simulink model "Wind_Turbine_test"  (R2023b)
settings: Solver=VariableStepAuto  StartTime=0.0  StopTime=1  RelTol=1e-3
model workspace (MAT data in the model file):
  Compensation_Ki = 30
  Compensation_Kp = 3
  DC_Ki = 400
  DC_Kp = 8
  F = 0.01
  Flux_min = 0.5
  Grid_Freq_PWM = 2700
  Grid_Ireg_Ki = 5
  Grid_Ireg_Kp = 0.83
  Grid_Ireg_lim = 1.1
  Grid_Modindex_Upper = 1.1
  Grid_conv_Imax = 0.8
  H = 0.685
  Idref_max = 0.9
  Iqref_Tc = 0.3
  Ki_Var = 0.05
  Ki_Vreg = 20
  Ksh = 1.1
  L_pu = 0.3
  Llr = 0.16
  Lls = 0.18
  Lm = 2.9
  P_mech = 1080000
  Pitch_Ki = 0
  Pitch_Kp = 150
  Pitch_Max = 27
  Pitch_Tc = 0.01
  Pitch_rate = 10
  Q_Filt = 50
  R_pu = 0.003
  Rotor_Freq_PWM = 1620
  Rotor_Ireg_Ki = 8
  Rotor_Ireg_Kp = 0.6
  Rotor_Ireg_lim = 0.1
  Rotor_Modindex_Upper = 2
  Rr = 0.016
  Rs = 0.023
  T_set = 0.0001
  Tp = 5e-05
  Ts = 5e-06
  Var_C_Filt = 720000
  Var_reg_max = 1.1
  Var_reg_min = 0.9
  WT_Coeff = [0.645 116 0.4 5 21 0.00912 0.08 0.035]
  WT_H = 4.32
  WT_IGBTRon = 5.931
  WT_Param = [91.204 10143]
  Wind_Freq_Filt = 10000
  Wind_Freq_nom = 60
  Wind_P_nom = 1200000
  Wind_Rotor_V_nom = 1950
  Wind_V_nom = 500
  Zeta_Filt = 0.707106781187
  init = [-0.2 0 0 0 0 0 0 0]
  p = 3
  torque0 = 0.83
  v_Ki = 0.1
  v_Kp = 3.6
  v_Max = 1.2
  v_Min = 0.7
  v_T = 5
  vreg_max = 1
  wind_VDC_nom = 1150
  wt0 = 1.2
undefined symbols (not defined in the file): D1, D11, Delta, DiscIntNeverNeededParam, P, Q
libraries: powerlib_extras x144, simulink_extras x24, spsThreePhaseVIMeasurementLib x13, spsThreePhaseTransformerTwoWindingsLib x11, spsSeriesRLCBranchLib x9, spsPWMGenerator2LevelLib x8, spsUniversalBridgeLib x8, spsThreePhaseSeriesRLCLoadLib x6, spsThreePhasePISectionLineLib x5, spsGroundLib x5, spsLoadFlowBusLib x4, spsAsynchronousMachinepuUnitsLib x4
(part 3 of 9)

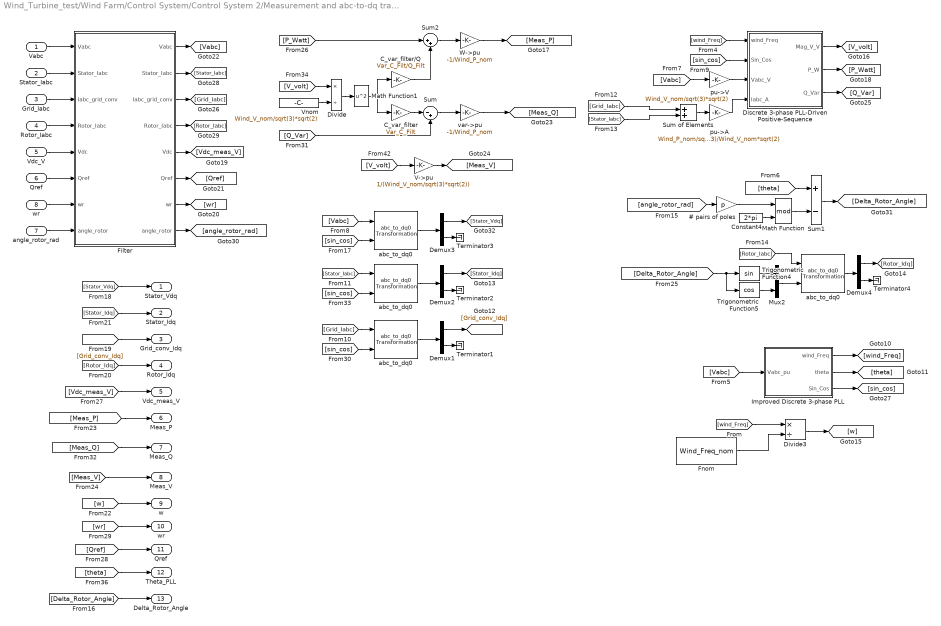
== system Wind_Turbine_test/Wind Farm/Control System/Control System 2/Measurement and abc-to-dq transformation  ==
  Vabc : Inport
  Stator_Iabc : Inport  Port=2
  Grid_Iabc : Inport  Port=3
  Rotor_Iabc : Inport  Port=4
  Vdc_V : Inport  Port=5
  Qref : Inport  Port=6
  angle_rotor_rad : Inport  Port=7
  wr : Inport  Port=8
  "   abc_to_dq0    " : powerlib_extras/Measurements/abc_to_dq0 Transformation
  " Improved Discrete 3-phase PLL" : Subsystem  mask(Discrete 3-phase PLL){Fmin=0.75*Wind_Freq_nom, Par_Init=[0 Wind_Freq_nom], ParK=[5 3.2 1 50], Ts=Ts}
      mask prompts: Fmin "Minimum frequency (Hz):"; Par_Init "Initial inputs:[ Phase(degrees)   Frequency(Hz) ]"; ParK "Regulator gains [ Kp1 Kp2  Ki1  Ki2 ]"; Ts "Sample time:"
      mask help:
      | This Phase Locked Loop (PLL) system can be used  to synchronize on a set of variable frequency, three-phase sinusoidal signals.
      |
      | Input 1: Vector containing the normalized
      |              three-phase signals [Va Vb Vc]
      | Output 1:  Measured frequency (Hz) = w/(2pi)
      | Output 2:  Ramp w.t   varying between  0 and 2*pi,
      | synchronized on zero crossings of the fundamental (positive-sequence) of phase A.
      | Output 3: Vector [sin(wt) cos(wt)]
      mask init:
      | Kp1=ParK(1);
      | Kp2=ParK(2);
      | Ki1=ParK(3);
      | Ki2=ParK(4);
      | Phase_Init=Par_Init(1);
      | Finit=Par_Init(2);
      | power_initmask();
      settings: OpenFcn=power_openblockproxy();
  # pairs of poles : Gain  Gain=p  SaturateOnIntegerOverflow=on  OutDataTypeStr=Inherit: Same as input  ParamDataTypeStr=Inherit: Same as input
  C_var_filter : Gain  Gain=Var_C_Filt  SaturateOnIntegerOverflow=on  OutDataTypeStr=Inherit: Same as input  ParamDataTypeStr=Inherit: Same as input
  C_var_filter/Q : Gain  Gain=Var_C_Filt/Q_Filt  SaturateOnIntegerOverflow=on  OutDataTypeStr=Inherit: Same as input  ParamDataTypeStr=Inherit: Same as input
  Constant4 : Constant  Value=2*pi
  Demux{1..4} (4 alike) : Demux  Outputs=[2 1]
      settings: DisplayOption=none
  "Discrete 3-phase PLL-Driven Positive-Sequence " : Subsystem  mask(Discrete 3-phase PLL-Driven Positive-Sequence Active & Reactive Power){Finit=Wind_Freq_nom, Fmin=Wind_Freq_nom*45/60, Par_Vinit=[Wind_V_nom/sqrt(3)*sqrt(2) 30], Par_Iinit=[Wind_P_nom/sqrt(3)/Wind_V_nom*sqrt(2) -10], Ts=Ts}
      mask prompts: Finit "Initial frequency (Hz):"; Fmin "Minimum frequency (Hz):"; Par_Vinit "Voltage initial input: [ Mag  Phase(Degrees) ]"; Par_Iinit "Current initial input: [ Mag  Phase(Degrees) ]"; Ts "Sample time:"
      mask help:
      | This discrete block measures the 3-phase active power P and reactive power Q  associated with a periodic set of 3-phase voltages and currents which may contain harmonics. P and Q are calculated by evaluating the fundamental values (positive-sequence) of the input voltages and currents with a running window over one cycle of the specified frequency (port Freq).
      |  Input port "Sin_Cos" (a two-dimension signal) provides the reference frame required for the computation.
      |
      | input 1: must give the frequency of the fundamental (Hz)
      | Input 2: must contain a  [sin(wt)  cos(wt)] two dimension signal , where w is the rotation speed (rad/s) of the reference frame used for the computation..
      | input 3: Vectorized 3-phase  instantaneous voltage (Vabc)
      | input 4: Vectorized 3-phase instantaneous current (Iabc)
      |
      | Output 1: Vector [Mag_V Mag_I] of the fundamental values (Magnitude) of the voltage & current (peak values of the positive-sequence)
      | Output 2: 3-phase PQ measurement vector [P(W) Q (var)] evaluated at the specified frequency. Current flowing into an RL circuit will produce  positive active and reactive powers.
      |
      | For the first cycle of simulation, the outputs are held constant using the values specified by the parameters "Initial input".
      | he value of the parameter "Minimum frequency" is used to determine the buffer size of the "Variable Transport Delay" block found inside this subsystem.
      mask init:
      | power_initmask();
      settings: OpenFcn=power_openblockproxy();
  Divide : Product  Inputs=*/
  Divide3 : Product  Inputs=*/
  Filter : Subsystem  mask{Freq=Wind_Freq_Filt, Zeta1=Zeta_Filt, Ts=Ts}
      mask prompts: Freq "Cut-off frequency (Hz):"; Zeta1 "Damping factor Zeta:"; Ts "Sample time"
  Fnom : Constant  Value=Wind_Freq_nom
  Math Function : Math  Operator=mod  SignedPower=on
  Math Function1 : Math  Operator=square  SignedPower=on
  Mux2 : Mux  Inputs=2
  Sum : Sum  Inputs=|-+
  Sum of Elements : Sum
  Sum1 : Sum  Inputs=+-  InputSameDT=on  SaturateOnIntegerOverflow=on  OutDataTypeStr=Inherit: Same as first input
  Sum2 : Sum  Inputs=|++
  Terminator{1..4} (4 alike) : Terminator
  Trigonometric Function4 : Trigonometry
  Trigonometric Function5 : Trigonometry  Operator=cos
  V->pu : Gain  Gain=1/(Wind_V_nom/sqrt(3)*sqrt(2))  SaturateOnIntegerOverflow=on  OutDataTypeStr=Inherit: Same as input  ParamDataTypeStr=Inherit: Same as input
  Vnom : Constant  Value=Wind_V_nom/sqrt(3)*sqrt(2)
  W->pu : Gain  Gain=-1/Wind_P_nom  SaturateOnIntegerOverflow=on  OutDataTypeStr=Inherit: Same as input  ParamDataTypeStr=Inherit: Same as input
  abc_to_dq0 : powerlib_extras/Measurements/abc_to_dq0 Transformation
  "abc_to_dq0 " : powerlib_extras/Measurements/abc_to_dq0 Transformation
  "abc_to_dq0  " : powerlib_extras/Measurements/abc_to_dq0 Transformation
  pu->A : Gain  Gain=Wind_P_nom/sqrt(3)/Wind_V_nom*sqrt(2)  SaturateOnIntegerOverflow=on  OutDataTypeStr=Inherit: Same as input  ParamDataTypeStr=Inherit: Same as input
  pu->V : Gain  Gain=Wind_V_nom/sqrt(3)*sqrt(2)  SaturateOnIntegerOverflow=on  OutDataTypeStr=Inherit: Same as input  ParamDataTypeStr=Inherit: Same as input
  "var->pu " : Gain  Gain=-1/Wind_P_nom  SaturateOnIntegerOverflow=on  OutDataTypeStr=Inherit: Same as input  ParamDataTypeStr=Inherit: Same as input
  Stator_Vdq : Outport  VectorParamsAs1DForOutWhenUnconnected=off
  Stator_Idq : Outport  Port=2  VectorParamsAs1DForOutWhenUnconnected=off
  Grid_conv_Idq : Outport  Port=3  VectorParamsAs1DForOutWhenUnconnected=off
  Rotor_Idq : Outport  Port=4  VectorParamsAs1DForOutWhenUnconnected=off
  Vdc_meas_V : Outport  Port=5  VectorParamsAs1DForOutWhenUnconnected=off
  Meas_P : Outport  Port=6  VectorParamsAs1DForOutWhenUnconnected=off
  Meas_Q : Outport  Port=7  VectorParamsAs1DForOutWhenUnconnected=off
  Meas_V : Outport  Port=8  VectorParamsAs1DForOutWhenUnconnected=off
  w : Outport  Port=9  VectorParamsAs1DForOutWhenUnconnected=off
  "wr " : Outport  Port=10  VectorParamsAs1DForOutWhenUnconnected=off
  "Qref " : Outport  Port=11  VectorParamsAs1DForOutWhenUnconnected=off
  Theta_PLL : Outport  Port=12  VectorParamsAs1DForOutWhenUnconnected=off
  Delta_Rotor_Angle : Outport  Port=13  VectorParamsAs1DForOutWhenUnconnected=off
  wires:
  Math Function/1 -> Sum1/2
  [wind_Freq] -> "Discrete 3-phase PLL-Driven Positive-Sequence "/1(wind_Freq)
  [P_Watt] -> Sum2/1
  [sin_cos] -> abc_to_dq0/2
  [Meas_Q] -> Meas_Q/1
  [Q_Var] -> Sum/2
  Math Function1/1 -> C_var_filter/Q/1, C_var_filter/1
  Sum of Elements/1 -> pu->A/1
  [Grid_Iabc] -> Sum of Elements/1
  [Grid_conv_Idq] -> Grid_conv_Idq/1
  Filter/6("Qref ") -> [Qref]
  W->pu/1 -> [Meas_P]
  [Stator_Idq] -> Stator_Idq/1
  "Discrete 3-phase PLL-Driven Positive-Sequence "/1(Mag_V_V) -> [V_volt]
  Demux1/2 -> Terminator1/1
  [wr] -> "wr "/1
  Filter/3("Iabc_grid_conv ") -> [Grid_Iabc]
  Filter/2("Stator_Iabc ") -> [Stator_Iabc]
  [Meas_P] -> Meas_P/1
  [Delta_Rotor_Angle] -> Trigonometric Function4/1, Trigonometric Function5/1
  Vnom/1 -> Divide/2
  [w] -> w/1
  "var->pu "/1 -> [Meas_Q]
  Sum2/1 -> W->pu/1
  [wind_Freq] -> Divide3/1
  [Delta_Rotor_Angle] -> Delta_Rotor_Angle/1
  Vdc_V/1 -> Filter/5(Vdc)
  "Discrete 3-phase PLL-Driven Positive-Sequence "/3(Q_Var) -> [Q_Var]
  [Vabc] -> pu->V/1
  wr/1 -> Filter/7(wr)
  Fnom/1 -> Divide3/2
  [Vabc] -> " Improved Discrete 3-phase PLL"/1(Vabc_pu)
  "Discrete 3-phase PLL-Driven Positive-Sequence "/2(P_W) -> [P_Watt]
  Trigonometric Function5/1 -> Mux2/2
  [sin_cos] -> "abc_to_dq0 "/2
  [V_volt] -> Divide/1
  Demux3/2 -> Terminator3/1
  Filter/5("Vdc ") -> [Vdc_meas_V]
  Filter/1("Vabc ") -> [Vabc]
  [sin_cos] -> "abc_to_dq0  "/2
  angle_rotor_rad/1 -> Filter/8(angle_rotor)
  "   abc_to_dq0    "/1 -> Demux4/1
  Divide3/1 -> [w]
  Divide/1 -> Math Function1/1
  # pairs of poles/1 -> Math Function/1
  [Stator_Iabc] -> "abc_to_dq0 "/1
  Filter/8("angle_rotor ") -> [angle_rotor_rad]
  Sum/1 -> "var->pu "/1
  [Stator_Vdq] -> Stator_Vdq/1
  Demux4/1 -> [Rotor_Idq]
  [Grid_Iabc] -> "abc_to_dq0  "/1
  [angle_rotor_rad] -> # pairs of poles/1
  Mux2/1 -> "   abc_to_dq0    "/2
  Demux2/2 -> Terminator2/1
  [V_volt] -> V->pu/1
  [Rotor_Iabc] -> "   abc_to_dq0    "/1
  Demux1/1 -> [Grid_conv_Idq]
  Filter/7("wr ") -> [wr]
  [Meas_V] -> Meas_V/1
  [Rotor_Idq] -> Rotor_Idq/1
  Constant4/1 -> Math Function/2
  Demux4/2 -> Terminator4/1
  [sin_cos] -> "Discrete 3-phase PLL-Driven Positive-Sequence "/2(Sin_Cos)
  Qref/1 -> Filter/6(Qref)
  Trigonometric Function4/1 -> Mux2/1
  [Vabc] -> abc_to_dq0/1
  Vabc/1 -> Filter/1(Vabc)
  Rotor_Iabc/1 -> Filter/4(Rotor_Iabc)
  [Qref] -> "Qref "/1
  C_var_filter/Q/1 -> Sum2/2
  Grid_Iabc/1 -> Filter/3(Iabc_grid_conv)
  " Improved Discrete 3-phase PLL"/3(Sin_Cos) -> [sin_cos]
  abc_to_dq0/1 -> Demux3/1
  Stator_Iabc/1 -> Filter/2(Stator_Iabc)
  V->pu/1 -> [Meas_V]
  "abc_to_dq0  "/1 -> Demux1/1
  Demux3/1 -> [Stator_Vdq]
  " Improved Discrete 3-phase PLL"/1(wind_Freq) -> [wind_Freq]
  [theta] -> Theta_PLL/1
  [Vdc_meas_V] -> Vdc_meas_V/1
  Filter/4("Rotor_Iabc ") -> [Rotor_Iabc]
  Sum1/1 -> [Delta_Rotor_Angle]
  "abc_to_dq0 "/1 -> Demux2/1
  [Stator_Iabc] -> Sum of Elements/2
  C_var_filter/1 -> Sum/1
  pu->V/1 -> "Discrete 3-phase PLL-Driven Positive-Sequence "/3(Vabc_V)
  Demux2/1 -> [Stator_Idq]
  [theta] -> Sum1/1
  " Improved Discrete 3-phase PLL"/2(theta) -> [theta]
  pu->A/1 -> "Discrete 3-phase PLL-Driven Positive-Sequence "/4(Iabc_A)

== system Wind_Turbine_test/Wind Farm/Control System/Control System 2/Rotor-side Control System ==
  Rotor_Idq : Inport
  wr : Inport  Port=2
  Vdc : Inport  Port=3
  Angle : Inport  Port=4
  Qref : Inport  Port=5
  Meas_Q : Inport  Port=6
  Meas_V : Inport  Port=7
  Stator_Vdq : Inport  Port=8
  w : Inport  Port=9
  Stator_Idq : Inport  Port=10
  Tem_cmd : Inport  Port=11
  Current Regulator : Subsystem
  "Electromagnetic Torque Controller " : Subsystem
  Gain : Gain  Gain=-1
  "Iqr, ref_limit" : Subsystem
  Modulation Index & Phase : Subsystem
  Rotor Control Voltage Converter : Subsystem
  Var Regulator : Subsystem
  Voltage Regulator : Subsystem
  Uctrl_rotor_conv : Outport  VectorParamsAs1DForOutWhenUnconnected=off
  wires:
  "Electromagnetic Torque Controller "/1(Rotor_Id_ref) -> Current Regulator/1(Rotor_Id_ref), "Iqr, ref_limit"/1(Rotor_Id_ref)
  Qref/1 -> Var Regulator/1(Qref)
  Meas_Q/1 -> Var Regulator/2(Meas_Q)
  Meas_V/1 -> Var Regulator/3(Meas_V)
  "Iqr, ref_limit"/1(Iqrlim) -> Voltage Regulator/1(Max), Gain/1
  Var Regulator/1(Out1) -> Voltage Regulator/3(In)
  Rotor_Idq/1 -> Current Regulator/2(Rotor_Idq)
  wr/1 -> Current Regulator/4(wr)
  Voltage Regulator/1(Iqr_ref) -> Current Regulator/3(Iqr_ref)
  Angle/1 -> Rotor Control Voltage Converter/3(Angle)
  Rotor Control Voltage Converter/1(Uctrl_rotor_conv) -> Uctrl_rotor_conv/1
  Vdc/1 -> Modulation Index & Phase/3(Vdc)
  Modulation Index & Phase/1(x1) -> Rotor Control Voltage Converter/1(x1)
  Modulation Index & Phase/2(y1) -> Rotor Control Voltage Converter/2(y1)
  Current Regulator/1(Rotor_conv_Vd) -> Modulation Index & Phase/1(x)
  Current Regulator/2(Rotor_conv_Vq) -> Modulation Index & Phase/2(y)
  Stator_Vdq/1 -> "Electromagnetic Torque Controller "/1(Stator_Vdq)
  w/1 -> "Electromagnetic Torque Controller "/2(w)
  Stator_Idq/1 -> "Electromagnetic Torque Controller "/3(Stator_Idq)
  Tem_cmd/1 -> "Electromagnetic Torque Controller "/4(Tem_cmd)
  Gain/1 -> Voltage Regulator/2(Min)

== system Wind_Turbine_test/Wind Farm/Control System/Control System 2/Speed & Pitch Control System ==
  wr1 : Inport
  Meas_P : Inport  Port=2
  0-inf : Saturate  UpperLimit=inf  LowerLimit=0
  0-pitch_max : Saturate  UpperLimit=Pitch_Max  LowerLimit=0
  "0-pitch_max " : Saturate  UpperLimit=Pitch_Max  LowerLimit=0
  Constant2 : Constant
  Discrete PI Controller : Subsystem  DialogController=POWERSYS.PowerSysDialog  mask(Discrete PI Controller){Kp=v_Kp, Ki=v_Ki, Par_Limits=[vreg_max 0], Init=0.7, Ts=Ts}
      mask prompts: Kp "Proportional gain (Kp):"; Ki "Integral gain (Ki):"; Par_Limits "Output limits: [ Upper   Lower ]"; Init "Output initial value:"; Ts "Sample time:"
      mask help: This block implements a discrete PI controller.
      mask init:
      | UpperLimit=Par_Limits(1);
      | LowerLimit=Par_Limits(2);
      | power_initmask();
      mask Help: This block is part of a subset of blocks in the Extras library that does not have documentation associated with it, other than the block mask description.
      mask Display: disp('PI');
  Discrete PI Controller1 : powerlib_extras/Discrete  Control Blocks/Discrete PI Controller  Kp=Compensation_Kp  Ki=Compensation_Ki  Par_Limits=[Pitch_Max 0]  Init=0  Ts=Ts
  Gain2 : Gain  Gain=Pitch_Kp  SaturateOnIntegerOverflow=on  OutDataTypeStr=Inherit: Same as input  ParamDataTypeStr=Inherit: Same as input
  Rate Limiter   1 : RateLimiter  RisingSlewLimit=Pitch_rate  FallingSlewLimit=-Pitch_rate
  Saturation : Saturate  UpperLimit=v_Max  LowerLimit=v_Min
  Sum : Sum  Inputs=-+  SaturateOnIntegerOverflow=on
  Sum1 : Sum  Inputs=|+-
  Sum2 : Sum  Inputs=|+-  SaturateOnIntegerOverflow=on
  Sum3 : Sum  Inputs=|++
  Switch : Switch  Threshold=0.75  SaturateOnIntegerOverflow=off  InputSameDT=off
  Tracking Curve : Fcn  Expr=-0.67*u(1)^2+1.42*u(1)+0.51
  pu_elec->pu_mec : Gain  Gain=Wind_P_nom/P_mech
  t=Pitch_time_constant : powerlib_extras/Discrete  Control Blocks/Discrete 1st-Order Filter  FilterType=Lowpass  Tc=Pitch_Tc  Ts=Ts  Initialize=on  Vac_Init=[0.8 -25 60]*0  Vdc_Init=0  PlotResponse=off  param1=[1 500 0.1]
  t=T_speed : powerlib_extras/Discrete  Control Blocks/Discrete 1st-Order Filter  FilterType=Lowpass  Tc=v_T  Ts=Ts  Initialize=on  Vac_Init=[0 0 0]  Vdc_Init=1-init(1)  PlotResponse=off  param1=[1 500 0.1]
  wref : Constant  Value=1.2
  Tem_cmd : Outport  VectorParamsAs1DForOutWhenUnconnected=off
  Pitch (deg) : Outport  Port=2  VectorParamsAs1DForOutWhenUnconnected=off
  wires:
  Rate Limiter   1/1 -> "0-pitch_max "/1
  Switch/1 -> Saturation/1
  Sum3/1 -> Rate Limiter   1/1
  Sum1/1 -> Discrete PI Controller/1(Error)
  Saturation/1 -> t=T_speed/1
  Constant2/1 -> Sum2/2  "Pref"
  Discrete PI Controller1/1 -> Sum3/2
  Meas_P/1 -> 0-inf/1
  t=T_speed/1 -> Sum/1, Sum1/2  "wref"
  0-inf/1 -> pu_elec->pu_mec/1
  wr1/1 -> Sum/2, Sum1/1
  wref/1 -> Switch/1
  0-pitch_max/1 -> Sum3/1
  Discrete PI Controller/1(Out) -> Tem_cmd/1
  t=Pitch_time_constant/1 -> Pitch (deg)/1
  Sum2/1 -> Discrete PI Controller1/1
  Gain2/1 -> 0-pitch_max/1
  pu_elec->pu_mec/1 -> Switch/2, Tracking Curve/1, Sum2/1
  "0-pitch_max "/1 -> t=Pitch_time_constant/1
  Sum/1 -> Gain2/1
  Tracking Curve/1 -> Switch/3

== system Wind_Turbine_test/Wind Farm/Control System/Control System 3/Grid-side Control System ==
  note: Required value for modulation index "m" to obtain 1 pu generated voltage by the converter:
  note: m = Vnom * 2*sqrt(2/3) / Vdc
  note: Where Vnom = RMS ph-ph nominal voltage
  Stator_Vdq : Inport
  Iq_ref : Inport  Port=2
  Vdc : Inport  Port=3
  Grid_conv_Idq : Inport  Port=4
  Theta_PLL : Inport  Port=5
  w : Inport  Port=6
  Current Regulator : Subsystem
  Grid Voltage Converter : Subsystem
  Modulation : Subsystem
  VDC Regulator : Subsystem
  Grid_conv_V : Outport  VectorParamsAs1DForOutWhenUnconnected=off
  wires:
  Current Regulator/1(Grid_conv_Vd) -> Modulation/1(x)
  Current Regulator/2(Grid_conv_Vq) -> Modulation/2(y)
  Grid Voltage Converter/1(Grid_conv_V) -> Grid_conv_V/1
  Theta_PLL/1 -> Grid Voltage Converter/2(Theta_PLL)
  VDC Regulator/1(Out1) -> Current Regulator/2(In2)
  Iq_ref/1 -> VDC Regulator/1(Iq_ref)
  Grid_conv_Idq/1 -> Current Regulator/3(Grid_conv_Idq)
  Stator_Vdq/1 -> Current Regulator/1(Stator_Vdq)
  w/1 -> Current Regulator/4(w)
  Modulation/1(Vdq0) -> Grid Voltage Converter/1(dq0)
  Vdc/1 -> VDC Regulator/2(Vdc)

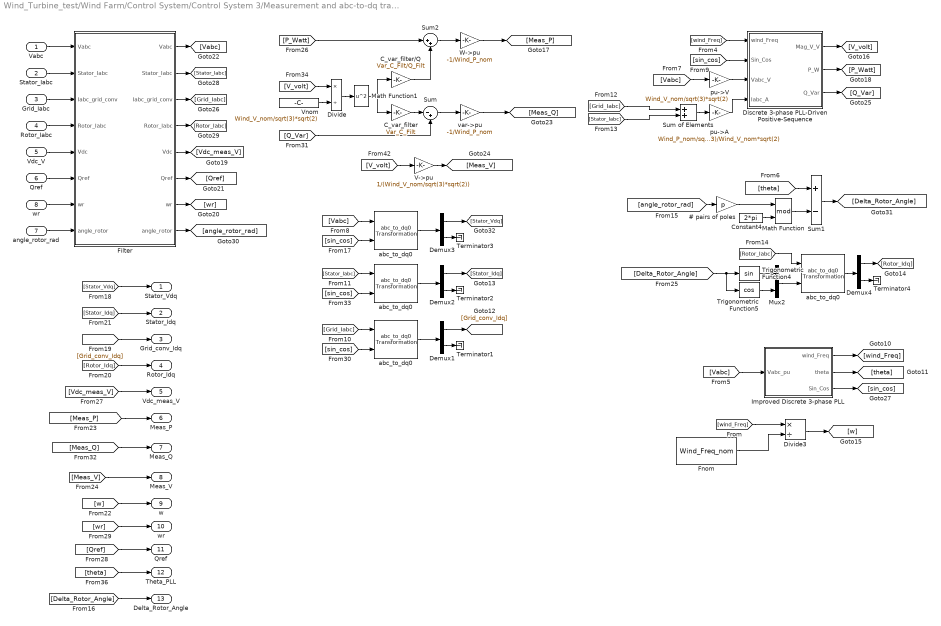
== system Wind_Turbine_test/Wind Farm/Control System/Control System 3/Measurement and abc-to-dq transformation  ==
  Vabc : Inport
  Stator_Iabc : Inport  Port=2
  Grid_Iabc : Inport  Port=3
  Rotor_Iabc : Inport  Port=4
  Vdc_V : Inport  Port=5
  Qref : Inport  Port=6
  angle_rotor_rad : Inport  Port=7
  wr : Inport  Port=8
  "   abc_to_dq0    " : powerlib_extras/Measurements/abc_to_dq0 Transformation
  " Improved Discrete 3-phase PLL" : Subsystem  mask(Discrete 3-phase PLL){Fmin=0.75*Wind_Freq_nom, Par_Init=[0 Wind_Freq_nom], ParK=[5 3.2 1 50], Ts=Ts}
      mask prompts: Fmin "Minimum frequency (Hz):"; Par_Init "Initial inputs:[ Phase(degrees)   Frequency(Hz) ]"; ParK "Regulator gains [ Kp1 Kp2  Ki1  Ki2 ]"; Ts "Sample time:"
      mask help:
      | This Phase Locked Loop (PLL) system can be used  to synchronize on a set of variable frequency, three-phase sinusoidal signals.
      |
      | Input 1: Vector containing the normalized
      |              three-phase signals [Va Vb Vc]
      | Output 1:  Measured frequency (Hz) = w/(2pi)
      | Output 2:  Ramp w.t   varying between  0 and 2*pi,
      | synchronized on zero crossings of the fundamental (positive-sequence) of phase A.
      | Output 3: Vector [sin(wt) cos(wt)]
      mask init:
      | Kp1=ParK(1);
      | Kp2=ParK(2);
      | Ki1=ParK(3);
      | Ki2=ParK(4);
      | Phase_Init=Par_Init(1);
      | Finit=Par_Init(2);
      | power_initmask();
      settings: OpenFcn=power_openblockproxy();
  # pairs of poles : Gain  Gain=p  SaturateOnIntegerOverflow=on  OutDataTypeStr=Inherit: Same as input  ParamDataTypeStr=Inherit: Same as input
  C_var_filter : Gain  Gain=Var_C_Filt  SaturateOnIntegerOverflow=on  OutDataTypeStr=Inherit: Same as input  ParamDataTypeStr=Inherit: Same as input
  C_var_filter/Q : Gain  Gain=Var_C_Filt/Q_Filt  SaturateOnIntegerOverflow=on  OutDataTypeStr=Inherit: Same as input  ParamDataTypeStr=Inherit: Same as input
  Constant4 : Constant  Value=2*pi
  Demux{1..4} (4 alike) : Demux  Outputs=[2 1]
      settings: DisplayOption=none
  "Discrete 3-phase PLL-Driven Positive-Sequence " : Subsystem  mask(Discrete 3-phase PLL-Driven Positive-Sequence Active & Reactive Power){Finit=Wind_Freq_nom, Fmin=Wind_Freq_nom*45/60, Par_Vinit=[Wind_V_nom/sqrt(3)*sqrt(2) 30], Par_Iinit=[Wind_P_nom/sqrt(3)/Wind_V_nom*sqrt(2) -10], Ts=Ts}
      mask prompts: Finit "Initial frequency (Hz):"; Fmin "Minimum frequency (Hz):"; Par_Vinit "Voltage initial input: [ Mag  Phase(Degrees) ]"; Par_Iinit "Current initial input: [ Mag  Phase(Degrees) ]"; Ts "Sample time:"
      mask help:
      | This discrete block measures the 3-phase active power P and reactive power Q  associated with a periodic set of 3-phase voltages and currents which may contain harmonics. P and Q are calculated by evaluating the fundamental values (positive-sequence) of the input voltages and currents with a running window over one cycle of the specified frequency (port Freq).
      |  Input port "Sin_Cos" (a two-dimension signal) provides the reference frame required for the computation.
      |
      | input 1: must give the frequency of the fundamental (Hz)
      | Input 2: must contain a  [sin(wt)  cos(wt)] two dimension signal , where w is the rotation speed (rad/s) of the reference frame used for the computation..
      | input 3: Vectorized 3-phase  instantaneous voltage (Vabc)
      | input 4: Vectorized 3-phase instantaneous current (Iabc)
      |
      | Output 1: Vector [Mag_V Mag_I] of the fundamental values (Magnitude) of the voltage & current (peak values of the positive-sequence)
      | Output 2: 3-phase PQ measurement vector [P(W) Q (var)] evaluated at the specified frequency. Current flowing into an RL circuit will produce  positive active and reactive powers.
      |
      | For the first cycle of simulation, the outputs are held constant using the values specified by the parameters "Initial input".
      | he value of the parameter "Minimum frequency" is used to determine the buffer size of the "Variable Transport Delay" block found inside this subsystem.
      mask init:
      | power_initmask();
      settings: OpenFcn=power_openblockproxy();
  Divide : Product  Inputs=*/
  Divide3 : Product  Inputs=*/
  Filter : Subsystem  mask{Freq=Wind_Freq_Filt, Zeta1=Zeta_Filt, Ts=Ts}
      mask prompts: Freq "Cut-off frequency (Hz):"; Zeta1 "Damping factor Zeta:"; Ts "Sample time"
  Fnom : Constant  Value=Wind_Freq_nom
  Math Function : Math  Operator=mod  SignedPower=on
  Math Function1 : Math  Operator=square  SignedPower=on
  Mux2 : Mux  Inputs=2
  Sum : Sum  Inputs=|-+
  Sum of Elements : Sum
  Sum1 : Sum  Inputs=+-  InputSameDT=on  SaturateOnIntegerOverflow=on  OutDataTypeStr=Inherit: Same as first input
  Sum2 : Sum  Inputs=|++
  Terminator{1..4} (4 alike) : Terminator
  Trigonometric Function4 : Trigonometry
  Trigonometric Function5 : Trigonometry  Operator=cos
  V->pu : Gain  Gain=1/(Wind_V_nom/sqrt(3)*sqrt(2))  SaturateOnIntegerOverflow=on  OutDataTypeStr=Inherit: Same as input  ParamDataTypeStr=Inherit: Same as input
  Vnom : Constant  Value=Wind_V_nom/sqrt(3)*sqrt(2)
  W->pu : Gain  Gain=-1/Wind_P_nom  SaturateOnIntegerOverflow=on  OutDataTypeStr=Inherit: Same as input  ParamDataTypeStr=Inherit: Same as input
  abc_to_dq0 : powerlib_extras/Measurements/abc_to_dq0 Transformation
  "abc_to_dq0 " : powerlib_extras/Measurements/abc_to_dq0 Transformation
  "abc_to_dq0  " : powerlib_extras/Measurements/abc_to_dq0 Transformation
  pu->A : Gain  Gain=Wind_P_nom/sqrt(3)/Wind_V_nom*sqrt(2)  SaturateOnIntegerOverflow=on  OutDataTypeStr=Inherit: Same as input  ParamDataTypeStr=Inherit: Same as input
  pu->V : Gain  Gain=Wind_V_nom/sqrt(3)*sqrt(2)  SaturateOnIntegerOverflow=on  OutDataTypeStr=Inherit: Same as input  ParamDataTypeStr=Inherit: Same as input
  "var->pu " : Gain  Gain=-1/Wind_P_nom  SaturateOnIntegerOverflow=on  OutDataTypeStr=Inherit: Same as input  ParamDataTypeStr=Inherit: Same as input
  Stator_Vdq : Outport  VectorParamsAs1DForOutWhenUnconnected=off
  Stator_Idq : Outport  Port=2  VectorParamsAs1DForOutWhenUnconnected=off
  Grid_conv_Idq : Outport  Port=3  VectorParamsAs1DForOutWhenUnconnected=off
  Rotor_Idq : Outport  Port=4  VectorParamsAs1DForOutWhenUnconnected=off
  Vdc_meas_V : Outport  Port=5  VectorParamsAs1DForOutWhenUnconnected=off
  Meas_P : Outport  Port=6  VectorParamsAs1DForOutWhenUnconnected=off
  Meas_Q : Outport  Port=7  VectorParamsAs1DForOutWhenUnconnected=off
  Meas_V : Outport  Port=8  VectorParamsAs1DForOutWhenUnconnected=off
  w : Outport  Port=9  VectorParamsAs1DForOutWhenUnconnected=off
  "wr " : Outport  Port=10  VectorParamsAs1DForOutWhenUnconnected=off
  "Qref " : Outport  Port=11  VectorParamsAs1DForOutWhenUnconnected=off
  Theta_PLL : Outport  Port=12  VectorParamsAs1DForOutWhenUnconnected=off
  Delta_Rotor_Angle : Outport  Port=13  VectorParamsAs1DForOutWhenUnconnected=off
  wires:
  Math Function/1 -> Sum1/2
  [wind_Freq] -> "Discrete 3-phase PLL-Driven Positive-Sequence "/1(wind_Freq)
  [P_Watt] -> Sum2/1
  [sin_cos] -> abc_to_dq0/2
  [Meas_Q] -> Meas_Q/1
  [Q_Var] -> Sum/2
  Math Function1/1 -> C_var_filter/Q/1, C_var_filter/1
  Sum of Elements/1 -> pu->A/1
  [Grid_Iabc] -> Sum of Elements/1
  [Grid_conv_Idq] -> Grid_conv_Idq/1
  Filter/6("Qref ") -> [Qref]
  W->pu/1 -> [Meas_P]
  [Stator_Idq] -> Stator_Idq/1
  "Discrete 3-phase PLL-Driven Positive-Sequence "/1(Mag_V_V) -> [V_volt]
  Demux1/2 -> Terminator1/1
  [wr] -> "wr "/1
  Filter/3("Iabc_grid_conv ") -> [Grid_Iabc]
  Filter/2("Stator_Iabc ") -> [Stator_Iabc]
  [Meas_P] -> Meas_P/1
  [Delta_Rotor_Angle] -> Trigonometric Function4/1, Trigonometric Function5/1
  Vnom/1 -> Divide/2
  [w] -> w/1
  "var->pu "/1 -> [Meas_Q]
  Sum2/1 -> W->pu/1
  [wind_Freq] -> Divide3/1
  [Delta_Rotor_Angle] -> Delta_Rotor_Angle/1
  Vdc_V/1 -> Filter/5(Vdc)
  "Discrete 3-phase PLL-Driven Positive-Sequence "/3(Q_Var) -> [Q_Var]
  [Vabc] -> pu->V/1
  wr/1 -> Filter/7(wr)
  Fnom/1 -> Divide3/2
  [Vabc] -> " Improved Discrete 3-phase PLL"/1(Vabc_pu)
  "Discrete 3-phase PLL-Driven Positive-Sequence "/2(P_W) -> [P_Watt]
  Trigonometric Function5/1 -> Mux2/2
  [sin_cos] -> "abc_to_dq0 "/2
  [V_volt] -> Divide/1
  Demux3/2 -> Terminator3/1
  Filter/5("Vdc ") -> [Vdc_meas_V]
  Filter/1("Vabc ") -> [Vabc]
  [sin_cos] -> "abc_to_dq0  "/2
  angle_rotor_rad/1 -> Filter/8(angle_rotor)
  "   abc_to_dq0    "/1 -> Demux4/1
  Divide3/1 -> [w]
  Divide/1 -> Math Function1/1
  # pairs of poles/1 -> Math Function/1
  [Stator_Iabc] -> "abc_to_dq0 "/1
  Filter/8("angle_rotor ") -> [angle_rotor_rad]
  Sum/1 -> "var->pu "/1
  [Stator_Vdq] -> Stator_Vdq/1
  Demux4/1 -> [Rotor_Idq]
  [Grid_Iabc] -> "abc_to_dq0  "/1
  [angle_rotor_rad] -> # pairs of poles/1
  Mux2/1 -> "   abc_to_dq0    "/2
  Demux2/2 -> Terminator2/1
  [V_volt] -> V->pu/1
  [Rotor_Iabc] -> "   abc_to_dq0    "/1
  Demux1/1 -> [Grid_conv_Idq]
  Filter/7("wr ") -> [wr]
  [Meas_V] -> Meas_V/1
  [Rotor_Idq] -> Rotor_Idq/1
  Constant4/1 -> Math Function/2
  Demux4/2 -> Terminator4/1
  [sin_cos] -> "Discrete 3-phase PLL-Driven Positive-Sequence "/2(Sin_Cos)
  Qref/1 -> Filter/6(Qref)
  Trigonometric Function4/1 -> Mux2/1
  [Vabc] -> abc_to_dq0/1
  Vabc/1 -> Filter/1(Vabc)
  Rotor_Iabc/1 -> Filter/4(Rotor_Iabc)
  [Qref] -> "Qref "/1
  C_var_filter/Q/1 -> Sum2/2
  Grid_Iabc/1 -> Filter/3(Iabc_grid_conv)
  " Improved Discrete 3-phase PLL"/3(Sin_Cos) -> [sin_cos]
  abc_to_dq0/1 -> Demux3/1
  Stator_Iabc/1 -> Filter/2(Stator_Iabc)
  V->pu/1 -> [Meas_V]
  "abc_to_dq0  "/1 -> Demux1/1
  Demux3/1 -> [Stator_Vdq]
  " Improved Discrete 3-phase PLL"/1(wind_Freq) -> [wind_Freq]
  [theta] -> Theta_PLL/1
  [Vdc_meas_V] -> Vdc_meas_V/1
  Filter/4("Rotor_Iabc ") -> [Rotor_Iabc]
  Sum1/1 -> [Delta_Rotor_Angle]
  "abc_to_dq0 "/1 -> Demux2/1
  [Stator_Iabc] -> Sum of Elements/2
  C_var_filter/1 -> Sum/1
  pu->V/1 -> "Discrete 3-phase PLL-Driven Positive-Sequence "/3(Vabc_V)
  Demux2/1 -> [Stator_Idq]
  [theta] -> Sum1/1
  " Improved Discrete 3-phase PLL"/2(theta) -> [theta]
  pu->A/1 -> "Discrete 3-phase PLL-Driven Positive-Sequence "/4(Iabc_A)

== system Wind_Turbine_test/Wind Farm/Control System/Control System 3/Rotor-side Control System ==
  Rotor_Idq : Inport
  wr : Inport  Port=2
  Vdc : Inport  Port=3
  Angle : Inport  Port=4
  Qref : Inport  Port=5
  Meas_Q : Inport  Port=6
  Meas_V : Inport  Port=7
  Stator_Vdq : Inport  Port=8
  w : Inport  Port=9
  Stator_Idq : Inport  Port=10
  Tem_cmd : Inport  Port=11
  Current Regulator : Subsystem
  "Electromagnetic Torque Controller " : Subsystem
  Gain : Gain  Gain=-1
  "Iqr, ref_limit" : Subsystem
  Modulation Index & Phase : Subsystem
  Rotor Control Voltage Converter : Subsystem
  Var Regulator : Subsystem
  Voltage Regulator : Subsystem
  Uctrl_rotor_conv : Outport  VectorParamsAs1DForOutWhenUnconnected=off
  wires:
  "Electromagnetic Torque Controller "/1(Rotor_Id_ref) -> Current Regulator/1(Rotor_Id_ref), "Iqr, ref_limit"/1(Rotor_Id_ref)
  Qref/1 -> Var Regulator/1(Qref)
  Meas_Q/1 -> Var Regulator/2(Meas_Q)
  Meas_V/1 -> Var Regulator/3(Meas_V)
  "Iqr, ref_limit"/1(Iqrlim) -> Voltage Regulator/1(Max), Gain/1
  Var Regulator/1(Out1) -> Voltage Regulator/3(In)
  Rotor_Idq/1 -> Current Regulator/2(Rotor_Idq)
  wr/1 -> Current Regulator/4(wr)
  Voltage Regulator/1(Iqr_ref) -> Current Regulator/3(Iqr_ref)
  Angle/1 -> Rotor Control Voltage Converter/3(Angle)
  Rotor Control Voltage Converter/1(Uctrl_rotor_conv) -> Uctrl_rotor_conv/1
  Vdc/1 -> Modulation Index & Phase/3(Vdc)
  Modulation Index & Phase/1(x1) -> Rotor Control Voltage Converter/1(x1)
  Modulation Index & Phase/2(y1) -> Rotor Control Voltage Converter/2(y1)
  Current Regulator/1(Rotor_conv_Vd) -> Modulation Index & Phase/1(x)
  Current Regulator/2(Rotor_conv_Vq) -> Modulation Index & Phase/2(y)
  Stator_Vdq/1 -> "Electromagnetic Torque Controller "/1(Stator_Vdq)
  w/1 -> "Electromagnetic Torque Controller "/2(w)
  Stator_Idq/1 -> "Electromagnetic Torque Controller "/3(Stator_Idq)
  Tem_cmd/1 -> "Electromagnetic Torque Controller "/4(Tem_cmd)
  Gain/1 -> Voltage Regulator/2(Min)

== system Wind_Turbine_test/Wind Farm/Control System/Control System 3/Speed & Pitch Control System ==
  wr1 : Inport
  Meas_P : Inport  Port=2
  0-inf : Saturate  UpperLimit=inf  LowerLimit=0
  0-pitch_max : Saturate  UpperLimit=Pitch_Max  LowerLimit=0
  "0-pitch_max " : Saturate  UpperLimit=Pitch_Max  LowerLimit=0
  Constant2 : Constant
  Discrete PI Controller : Subsystem  DialogController=POWERSYS.PowerSysDialog  mask(Discrete PI Controller){Kp=v_Kp, Ki=v_Ki, Par_Limits=[vreg_max 0], Init=0.7, Ts=Ts}
      mask prompts: Kp "Proportional gain (Kp):"; Ki "Integral gain (Ki):"; Par_Limits "Output limits: [ Upper   Lower ]"; Init "Output initial value:"; Ts "Sample time:"
      mask help: This block implements a discrete PI controller.
      mask init:
      | UpperLimit=Par_Limits(1);
      | LowerLimit=Par_Limits(2);
      | power_initmask();
      mask Help: This block is part of a subset of blocks in the Extras library that does not have documentation associated with it, other than the block mask description.
      mask Display: disp('PI');
  Discrete PI Controller1 : powerlib_extras/Discrete  Control Blocks/Discrete PI Controller  Kp=Compensation_Kp  Ki=Compensation_Ki  Par_Limits=[Pitch_Max 0]  Init=0  Ts=Ts
  Gain2 : Gain  Gain=Pitch_Kp  SaturateOnIntegerOverflow=on  OutDataTypeStr=Inherit: Same as input  ParamDataTypeStr=Inherit: Same as input
  Rate Limiter   1 : RateLimiter  RisingSlewLimit=Pitch_rate  FallingSlewLimit=-Pitch_rate
  Saturation : Saturate  UpperLimit=v_Max  LowerLimit=v_Min
  Sum : Sum  Inputs=-+  SaturateOnIntegerOverflow=on
  Sum1 : Sum  Inputs=|+-
  Sum2 : Sum  Inputs=|+-  SaturateOnIntegerOverflow=on
  Sum3 : Sum  Inputs=|++
  Switch : Switch  Threshold=0.75  SaturateOnIntegerOverflow=off  InputSameDT=off
  Tracking Curve : Fcn  Expr=-0.67*u(1)^2+1.42*u(1)+0.51
  pu_elec->pu_mec : Gain  Gain=Wind_P_nom/P_mech
  t=Pitch_time_constant : powerlib_extras/Discrete  Control Blocks/Discrete 1st-Order Filter  FilterType=Lowpass  Tc=Pitch_Tc  Ts=Ts  Initialize=on  Vac_Init=[0.8 -25 60]*0  Vdc_Init=0  PlotResponse=off  param1=[1 500 0.1]
  t=T_speed : powerlib_extras/Discrete  Control Blocks/Discrete 1st-Order Filter  FilterType=Lowpass  Tc=v_T  Ts=Ts  Initialize=on  Vac_Init=[0 0 0]  Vdc_Init=1-init(1)  PlotResponse=off  param1=[1 500 0.1]
  wref : Constant  Value=1.2
  Tem_cmd : Outport  VectorParamsAs1DForOutWhenUnconnected=off
  Pitch (deg) : Outport  Port=2  VectorParamsAs1DForOutWhenUnconnected=off
  wires:
  Rate Limiter   1/1 -> "0-pitch_max "/1
  Switch/1 -> Saturation/1
  Sum3/1 -> Rate Limiter   1/1
  Sum1/1 -> Discrete PI Controller/1(Error)
  Saturation/1 -> t=T_speed/1
  Constant2/1 -> Sum2/2  "Pref"
  Discrete PI Controller1/1 -> Sum3/2
  Meas_P/1 -> 0-inf/1
  t=T_speed/1 -> Sum/1, Sum1/2  "wref"
  0-inf/1 -> pu_elec->pu_mec/1
  wr1/1 -> Sum/2, Sum1/1
  wref/1 -> Switch/1
  0-pitch_max/1 -> Sum3/1
  Discrete PI Controller/1(Out) -> Tem_cmd/1
  t=Pitch_time_constant/1 -> Pitch (deg)/1
  Sum2/1 -> Discrete PI Controller1/1
  Gain2/1 -> 0-pitch_max/1
  pu_elec->pu_mec/1 -> Switch/2, Tracking Curve/1, Sum2/1
  "0-pitch_max "/1 -> t=Pitch_time_constant/1
  Sum/1 -> Gain2/1
  Tracking Curve/1 -> Switch/3

== system Wind_Turbine_test/Wind Farm/Control System/Control System 4/Grid-side Control System ==
  note: Required value for modulation index "m" to obtain 1 pu generated voltage by the converter:
  note: m = Vnom * 2*sqrt(2/3) / Vdc
  note: Where Vnom = RMS ph-ph nominal voltage
  Stator_Vdq : Inport
  Iq_ref : Inport  Port=2
  Vdc : Inport  Port=3
  Grid_conv_Idq : Inport  Port=4
  Theta_PLL : Inport  Port=5
  w : Inport  Port=6
  Current Regulator : Subsystem
  Grid Voltage Converter : Subsystem
  Modulation : Subsystem
  VDC Regulator : Subsystem
  Grid_conv_V : Outport  VectorParamsAs1DForOutWhenUnconnected=off
  wires:
  Current Regulator/1(Grid_conv_Vd) -> Modulation/1(x)
  Current Regulator/2(Grid_conv_Vq) -> Modulation/2(y)
  Grid Voltage Converter/1(Grid_conv_V) -> Grid_conv_V/1
  Theta_PLL/1 -> Grid Voltage Converter/2(Theta_PLL)
  VDC Regulator/1(Out1) -> Current Regulator/2(In2)
  Iq_ref/1 -> VDC Regulator/1(Iq_ref)
  Grid_conv_Idq/1 -> Current Regulator/3(Grid_conv_Idq)
  Stator_Vdq/1 -> Current Regulator/1(Stator_Vdq)
  w/1 -> Current Regulator/4(w)
  Modulation/1(Vdq0) -> Grid Voltage Converter/1(dq0)
  Vdc/1 -> VDC Regulator/2(Vdc)

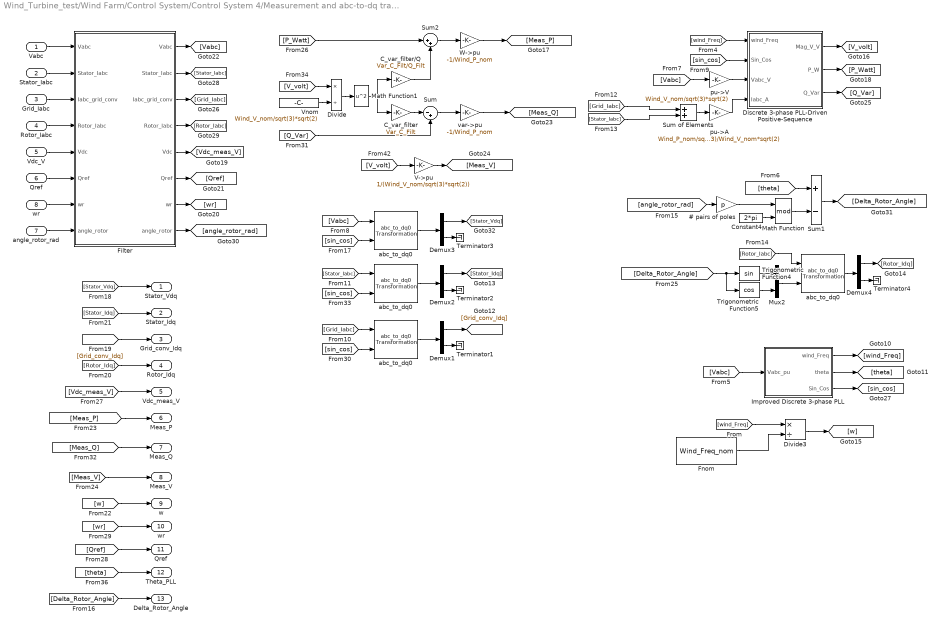
== system Wind_Turbine_test/Wind Farm/Control System/Control System 4/Measurement and abc-to-dq transformation  ==
  Vabc : Inport
  Stator_Iabc : Inport  Port=2
  Grid_Iabc : Inport  Port=3
  Rotor_Iabc : Inport  Port=4
  Vdc_V : Inport  Port=5
  Qref : Inport  Port=6
  angle_rotor_rad : Inport  Port=7
  wr : Inport  Port=8
  "   abc_to_dq0    " : powerlib_extras/Measurements/abc_to_dq0 Transformation
  " Improved Discrete 3-phase PLL" : Subsystem  mask(Discrete 3-phase PLL){Fmin=0.75*Wind_Freq_nom, Par_Init=[0 Wind_Freq_nom], ParK=[5 3.2 1 50], Ts=Ts}
      mask prompts: Fmin "Minimum frequency (Hz):"; Par_Init "Initial inputs:[ Phase(degrees)   Frequency(Hz) ]"; ParK "Regulator gains [ Kp1 Kp2  Ki1  Ki2 ]"; Ts "Sample time:"
      mask help:
      | This Phase Locked Loop (PLL) system can be used  to synchronize on a set of variable frequency, three-phase sinusoidal signals.
      |
      | Input 1: Vector containing the normalized
      |              three-phase signals [Va Vb Vc]
      | Output 1:  Measured frequency (Hz) = w/(2pi)
      | Output 2:  Ramp w.t   varying between  0 and 2*pi,
      | synchronized on zero crossings of the fundamental (positive-sequence) of phase A.
      | Output 3: Vector [sin(wt) cos(wt)]
      mask init:
      | Kp1=ParK(1);
      | Kp2=ParK(2);
      | Ki1=ParK(3);
      | Ki2=ParK(4);
      | Phase_Init=Par_Init(1);
      | Finit=Par_Init(2);
      | power_initmask();
      settings: OpenFcn=power_openblockproxy();
  # pairs of poles : Gain  Gain=p  SaturateOnIntegerOverflow=on  OutDataTypeStr=Inherit: Same as input  ParamDataTypeStr=Inherit: Same as input
  C_var_filter : Gain  Gain=Var_C_Filt  SaturateOnIntegerOverflow=on  OutDataTypeStr=Inherit: Same as input  ParamDataTypeStr=Inherit: Same as input
  C_var_filter/Q : Gain  Gain=Var_C_Filt/Q_Filt  SaturateOnIntegerOverflow=on  OutDataTypeStr=Inherit: Same as input  ParamDataTypeStr=Inherit: Same as input
  Constant4 : Constant  Value=2*pi
  Demux{1..4} (4 alike) : Demux  Outputs=[2 1]
      settings: DisplayOption=none
  "Discrete 3-phase PLL-Driven Positive-Sequence " : Subsystem  mask(Discrete 3-phase PLL-Driven Positive-Sequence Active & Reactive Power){Finit=Wind_Freq_nom, Fmin=Wind_Freq_nom*45/60, Par_Vinit=[Wind_V_nom/sqrt(3)*sqrt(2) 30], Par_Iinit=[Wind_P_nom/sqrt(3)/Wind_V_nom*sqrt(2) -10], Ts=Ts}
      mask prompts: Finit "Initial frequency (Hz):"; Fmin "Minimum frequency (Hz):"; Par_Vinit "Voltage initial input: [ Mag  Phase(Degrees) ]"; Par_Iinit "Current initial input: [ Mag  Phase(Degrees) ]"; Ts "Sample time:"
      mask help:
      | This discrete block measures the 3-phase active power P and reactive power Q  associated with a periodic set of 3-phase voltages and currents which may contain harmonics. P and Q are calculated by evaluating the fundamental values (positive-sequence) of the input voltages and currents with a running window over one cycle of the specified frequency (port Freq).
      |  Input port "Sin_Cos" (a two-dimension signal) provides the reference frame required for the computation.
      |
      | input 1: must give the frequency of the fundamental (Hz)
      | Input 2: must contain a  [sin(wt)  cos(wt)] two dimension signal , where w is the rotation speed (rad/s) of the reference frame used for the computation..
      | input 3: Vectorized 3-phase  instantaneous voltage (Vabc)
      | input 4: Vectorized 3-phase instantaneous current (Iabc)
      |
      | Output 1: Vector [Mag_V Mag_I] of the fundamental values (Magnitude) of the voltage & current (peak values of the positive-sequence)
      | Output 2: 3-phase PQ measurement vector [P(W) Q (var)] evaluated at the specified frequency. Current flowing into an RL circuit will produce  positive active and reactive powers.
      |
      | For the first cycle of simulation, the outputs are held constant using the values specified by the parameters "Initial input".
      | he value of the parameter "Minimum frequency" is used to determine the buffer size of the "Variable Transport Delay" block found inside this subsystem.
      mask init:
      | power_initmask();
      settings: OpenFcn=power_openblockproxy();
  Divide : Product  Inputs=*/
  Divide3 : Product  Inputs=*/
  Filter : Subsystem  mask{Freq=Wind_Freq_Filt, Zeta1=Zeta_Filt, Ts=Ts}
      mask prompts: Freq "Cut-off frequency (Hz):"; Zeta1 "Damping factor Zeta:"; Ts "Sample time"
  Fnom : Constant  Value=Wind_Freq_nom
  Math Function : Math  Operator=mod  SignedPower=on
  Math Function1 : Math  Operator=square  SignedPower=on
  Mux2 : Mux  Inputs=2
  Sum : Sum  Inputs=|-+
  Sum of Elements : Sum
  Sum1 : Sum  Inputs=+-  InputSameDT=on  SaturateOnIntegerOverflow=on  OutDataTypeStr=Inherit: Same as first input
  Sum2 : Sum  Inputs=|++
  Terminator{1..4} (4 alike) : Terminator
  Trigonometric Function4 : Trigonometry
  Trigonometric Function5 : Trigonometry  Operator=cos
  V->pu : Gain  Gain=1/(Wind_V_nom/sqrt(3)*sqrt(2))  SaturateOnIntegerOverflow=on  OutDataTypeStr=Inherit: Same as input  ParamDataTypeStr=Inherit: Same as input
  Vnom : Constant  Value=Wind_V_nom/sqrt(3)*sqrt(2)
  W->pu : Gain  Gain=-1/Wind_P_nom  SaturateOnIntegerOverflow=on  OutDataTypeStr=Inherit: Same as input  ParamDataTypeStr=Inherit: Same as input
  abc_to_dq0 : powerlib_extras/Measurements/abc_to_dq0 Transformation
  "abc_to_dq0 " : powerlib_extras/Measurements/abc_to_dq0 Transformation
  "abc_to_dq0  " : powerlib_extras/Measurements/abc_to_dq0 Transformation
  pu->A : Gain  Gain=Wind_P_nom/sqrt(3)/Wind_V_nom*sqrt(2)  SaturateOnIntegerOverflow=on  OutDataTypeStr=Inherit: Same as input  ParamDataTypeStr=Inherit: Same as input
  pu->V : Gain  Gain=Wind_V_nom/sqrt(3)*sqrt(2)  SaturateOnIntegerOverflow=on  OutDataTypeStr=Inherit: Same as input  ParamDataTypeStr=Inherit: Same as input
  "var->pu " : Gain  Gain=-1/Wind_P_nom  SaturateOnIntegerOverflow=on  OutDataTypeStr=Inherit: Same as input  ParamDataTypeStr=Inherit: Same as input
  Stator_Vdq : Outport  VectorParamsAs1DForOutWhenUnconnected=off
  Stator_Idq : Outport  Port=2  VectorParamsAs1DForOutWhenUnconnected=off
  Grid_conv_Idq : Outport  Port=3  VectorParamsAs1DForOutWhenUnconnected=off
  Rotor_Idq : Outport  Port=4  VectorParamsAs1DForOutWhenUnconnected=off
  Vdc_meas_V : Outport  Port=5  VectorParamsAs1DForOutWhenUnconnected=off
  Meas_P : Outport  Port=6  VectorParamsAs1DForOutWhenUnconnected=off
  Meas_Q : Outport  Port=7  VectorParamsAs1DForOutWhenUnconnected=off
  Meas_V : Outport  Port=8  VectorParamsAs1DForOutWhenUnconnected=off
  w : Outport  Port=9  VectorParamsAs1DForOutWhenUnconnected=off
  "wr " : Outport  Port=10  VectorParamsAs1DForOutWhenUnconnected=off
  "Qref " : Outport  Port=11  VectorParamsAs1DForOutWhenUnconnected=off
  Theta_PLL : Outport  Port=12  VectorParamsAs1DForOutWhenUnconnected=off
  Delta_Rotor_Angle : Outport  Port=13  VectorParamsAs1DForOutWhenUnconnected=off
  wires:
  Math Function/1 -> Sum1/2
  [wind_Freq] -> "Discrete 3-phase PLL-Driven Positive-Sequence "/1(wind_Freq)
  [P_Watt] -> Sum2/1
  [sin_cos] -> abc_to_dq0/2
  [Meas_Q] -> Meas_Q/1
  [Q_Var] -> Sum/2
  Math Function1/1 -> C_var_filter/Q/1, C_var_filter/1
  Sum of Elements/1 -> pu->A/1
  [Grid_Iabc] -> Sum of Elements/1
  [Grid_conv_Idq] -> Grid_conv_Idq/1
  Filter/6("Qref ") -> [Qref]
  W->pu/1 -> [Meas_P]
  [Stator_Idq] -> Stator_Idq/1
  "Discrete 3-phase PLL-Driven Positive-Sequence "/1(Mag_V_V) -> [V_volt]
  Demux1/2 -> Terminator1/1
  [wr] -> "wr "/1
  Filter/3("Iabc_grid_conv ") -> [Grid_Iabc]
  Filter/2("Stator_Iabc ") -> [Stator_Iabc]
  [Meas_P] -> Meas_P/1
  [Delta_Rotor_Angle] -> Trigonometric Function4/1, Trigonometric Function5/1
  Vnom/1 -> Divide/2
  [w] -> w/1
  "var->pu "/1 -> [Meas_Q]
  Sum2/1 -> W->pu/1
  [wind_Freq] -> Divide3/1
  [Delta_Rotor_Angle] -> Delta_Rotor_Angle/1
  Vdc_V/1 -> Filter/5(Vdc)
  "Discrete 3-phase PLL-Driven Positive-Sequence "/3(Q_Var) -> [Q_Var]
  [Vabc] -> pu->V/1
  wr/1 -> Filter/7(wr)
  Fnom/1 -> Divide3/2
  [Vabc] -> " Improved Discrete 3-phase PLL"/1(Vabc_pu)
  "Discrete 3-phase PLL-Driven Positive-Sequence "/2(P_W) -> [P_Watt]
  Trigonometric Function5/1 -> Mux2/2
  [sin_cos] -> "abc_to_dq0 "/2
  [V_volt] -> Divide/1
  Demux3/2 -> Terminator3/1
  Filter/5("Vdc ") -> [Vdc_meas_V]
  Filter/1("Vabc ") -> [Vabc]
  [sin_cos] -> "abc_to_dq0  "/2
  angle_rotor_rad/1 -> Filter/8(angle_rotor)
  "   abc_to_dq0    "/1 -> Demux4/1
  Divide3/1 -> [w]
  Divide/1 -> Math Function1/1
  # pairs of poles/1 -> Math Function/1
  [Stator_Iabc] -> "abc_to_dq0 "/1
  Filter/8("angle_rotor ") -> [angle_rotor_rad]
  Sum/1 -> "var->pu "/1
  [Stator_Vdq] -> Stator_Vdq/1
  Demux4/1 -> [Rotor_Idq]
  [Grid_Iabc] -> "abc_to_dq0  "/1
  [angle_rotor_rad] -> # pairs of poles/1
  Mux2/1 -> "   abc_to_dq0    "/2
  Demux2/2 -> Terminator2/1
  [V_volt] -> V->pu/1
  [Rotor_Iabc] -> "   abc_to_dq0    "/1
  Demux1/1 -> [Grid_conv_Idq]
  Filter/7("wr ") -> [wr]
  [Meas_V] -> Meas_V/1
  [Rotor_Idq] -> Rotor_Idq/1
  Constant4/1 -> Math Function/2
  Demux4/2 -> Terminator4/1
  [sin_cos] -> "Discrete 3-phase PLL-Driven Positive-Sequence "/2(Sin_Cos)
  Qref/1 -> Filter/6(Qref)
  Trigonometric Function4/1 -> Mux2/1
  [Vabc] -> abc_to_dq0/1
  Vabc/1 -> Filter/1(Vabc)
  Rotor_Iabc/1 -> Filter/4(Rotor_Iabc)
  [Qref] -> "Qref "/1
  C_var_filter/Q/1 -> Sum2/2
  Grid_Iabc/1 -> Filter/3(Iabc_grid_conv)
  " Improved Discrete 3-phase PLL"/3(Sin_Cos) -> [sin_cos]
  abc_to_dq0/1 -> Demux3/1
  Stator_Iabc/1 -> Filter/2(Stator_Iabc)
  V->pu/1 -> [Meas_V]
  "abc_to_dq0  "/1 -> Demux1/1
  Demux3/1 -> [Stator_Vdq]
  " Improved Discrete 3-phase PLL"/1(wind_Freq) -> [wind_Freq]
  [theta] -> Theta_PLL/1
  [Vdc_meas_V] -> Vdc_meas_V/1
  Filter/4("Rotor_Iabc ") -> [Rotor_Iabc]
  Sum1/1 -> [Delta_Rotor_Angle]
  "abc_to_dq0 "/1 -> Demux2/1
  [Stator_Iabc] -> Sum of Elements/2
  C_var_filter/1 -> Sum/1
  pu->V/1 -> "Discrete 3-phase PLL-Driven Positive-Sequence "/3(Vabc_V)
  Demux2/1 -> [Stator_Idq]
  [theta] -> Sum1/1
  " Improved Discrete 3-phase PLL"/2(theta) -> [theta]
  pu->A/1 -> "Discrete 3-phase PLL-Driven Positive-Sequence "/4(Iabc_A)

== system Wind_Turbine_test/Wind Farm/Control System/Control System 4/Rotor-side Control System ==
  Rotor_Idq : Inport
  wr : Inport  Port=2
  Vdc : Inport  Port=3
  Angle : Inport  Port=4
  Qref : Inport  Port=5
  Meas_Q : Inport  Port=6
  Meas_V : Inport  Port=7
  Stator_Vdq : Inport  Port=8
  w : Inport  Port=9
  Stator_Idq : Inport  Port=10
  Tem_cmd : Inport  Port=11
  Current Regulator : Subsystem
  "Electromagnetic Torque Controller " : Subsystem
  Gain : Gain  Gain=-1
  "Iqr, ref_limit" : Subsystem
  Modulation Index & Phase : Subsystem
  Rotor Control Voltage Converter : Subsystem
  Var Regulator : Subsystem
  Voltage Regulator : Subsystem
  Uctrl_rotor_conv : Outport  VectorParamsAs1DForOutWhenUnconnected=off
  wires:
  "Electromagnetic Torque Controller "/1(Rotor_Id_ref) -> Current Regulator/1(Rotor_Id_ref), "Iqr, ref_limit"/1(Rotor_Id_ref)
  Qref/1 -> Var Regulator/1(Qref)
  Meas_Q/1 -> Var Regulator/2(Meas_Q)
  Meas_V/1 -> Var Regulator/3(Meas_V)
  "Iqr, ref_limit"/1(Iqrlim) -> Voltage Regulator/1(Max), Gain/1
  Var Regulator/1(Out1) -> Voltage Regulator/3(In)
  Rotor_Idq/1 -> Current Regulator/2(Rotor_Idq)
  wr/1 -> Current Regulator/4(wr)
  Voltage Regulator/1(Iqr_ref) -> Current Regulator/3(Iqr_ref)
  Angle/1 -> Rotor Control Voltage Converter/3(Angle)
  Rotor Control Voltage Converter/1(Uctrl_rotor_conv) -> Uctrl_rotor_conv/1
  Vdc/1 -> Modulation Index & Phase/3(Vdc)
  Modulation Index & Phase/1(x1) -> Rotor Control Voltage Converter/1(x1)
  Modulation Index & Phase/2(y1) -> Rotor Control Voltage Converter/2(y1)
  Current Regulator/1(Rotor_conv_Vd) -> Modulation Index & Phase/1(x)
  Current Regulator/2(Rotor_conv_Vq) -> Modulation Index & Phase/2(y)
  Stator_Vdq/1 -> "Electromagnetic Torque Controller "/1(Stator_Vdq)
  w/1 -> "Electromagnetic Torque Controller "/2(w)
  Stator_Idq/1 -> "Electromagnetic Torque Controller "/3(Stator_Idq)
  Tem_cmd/1 -> "Electromagnetic Torque Controller "/4(Tem_cmd)
  Gain/1 -> Voltage Regulator/2(Min)

== system Wind_Turbine_test/Wind Farm/Control System/Control System 4/Speed & Pitch Control System ==
  wr1 : Inport
  Meas_P : Inport  Port=2
  0-inf : Saturate  UpperLimit=inf  LowerLimit=0
  0-pitch_max : Saturate  UpperLimit=Pitch_Max  LowerLimit=0
  "0-pitch_max " : Saturate  UpperLimit=Pitch_Max  LowerLimit=0
  Constant2 : Constant
  Discrete PI Controller : Subsystem  DialogController=POWERSYS.PowerSysDialog  mask(Discrete PI Controller){Kp=v_Kp, Ki=v_Ki, Par_Limits=[vreg_max 0], Init=0.7, Ts=Ts}
      mask prompts: Kp "Proportional gain (Kp):"; Ki "Integral gain (Ki):"; Par_Limits "Output limits: [ Upper   Lower ]"; Init "Output initial value:"; Ts "Sample time:"
      mask help: This block implements a discrete PI controller.
      mask init:
      | UpperLimit=Par_Limits(1);
      | LowerLimit=Par_Limits(2);
      | power_initmask();
      mask Help: This block is part of a subset of blocks in the Extras library that does not have documentation associated with it, other than the block mask description.
      mask Display: disp('PI');
  Discrete PI Controller1 : powerlib_extras/Discrete  Control Blocks/Discrete PI Controller  Kp=Compensation_Kp  Ki=Compensation_Ki  Par_Limits=[Pitch_Max 0]  Init=0  Ts=Ts
  Gain2 : Gain  Gain=Pitch_Kp  SaturateOnIntegerOverflow=on  OutDataTypeStr=Inherit: Same as input  ParamDataTypeStr=Inherit: Same as input
  Rate Limiter   1 : RateLimiter  RisingSlewLimit=Pitch_rate  FallingSlewLimit=-Pitch_rate
  Saturation : Saturate  UpperLimit=v_Max  LowerLimit=v_Min
  Sum : Sum  Inputs=-+  SaturateOnIntegerOverflow=on
  Sum1 : Sum  Inputs=|+-
  Sum2 : Sum  Inputs=|+-  SaturateOnIntegerOverflow=on
  Sum3 : Sum  Inputs=|++
  Switch : Switch  Threshold=0.75  SaturateOnIntegerOverflow=off  InputSameDT=off
  Tracking Curve : Fcn  Expr=-0.67*u(1)^2+1.42*u(1)+0.51
  pu_elec->pu_mec : Gain  Gain=Wind_P_nom/P_mech
  t=Pitch_time_constant : powerlib_extras/Discrete  Control Blocks/Discrete 1st-Order Filter  FilterType=Lowpass  Tc=Pitch_Tc  Ts=Ts  Initialize=on  Vac_Init=[0.8 -25 60]*0  Vdc_Init=0  PlotResponse=off  param1=[1 500 0.1]
  t=T_speed : powerlib_extras/Discrete  Control Blocks/Discrete 1st-Order Filter  FilterType=Lowpass  Tc=v_T  Ts=Ts  Initialize=on  Vac_Init=[0 0 0]  Vdc_Init=1-init(1)  PlotResponse=off  param1=[1 500 0.1]
  wref : Constant  Value=1.2
  Tem_cmd : Outport  VectorParamsAs1DForOutWhenUnconnected=off
  Pitch (deg) : Outport  Port=2  VectorParamsAs1DForOutWhenUnconnected=off
  wires:
  Rate Limiter   1/1 -> "0-pitch_max "/1
  Switch/1 -> Saturation/1
  Sum3/1 -> Rate Limiter   1/1
  Sum1/1 -> Discrete PI Controller/1(Error)
  Saturation/1 -> t=T_speed/1
  Constant2/1 -> Sum2/2  "Pref"
  Discrete PI Controller1/1 -> Sum3/2
  Meas_P/1 -> 0-inf/1
  t=T_speed/1 -> Sum/1, Sum1/2  "wref"
  0-inf/1 -> pu_elec->pu_mec/1
  wr1/1 -> Sum/2, Sum1/1
  wref/1 -> Switch/1
  0-pitch_max/1 -> Sum3/1
  Discrete PI Controller/1(Out) -> Tem_cmd/1
  t=Pitch_time_constant/1 -> Pitch (deg)/1
  Sum2/1 -> Discrete PI Controller1/1
  Gain2/1 -> 0-pitch_max/1
  pu_elec->pu_mec/1 -> Switch/2, Tracking Curve/1, Sum2/1
  "0-pitch_max "/1 -> t=Pitch_time_constant/1
  Sum/1 -> Gain2/1
  Tracking Curve/1 -> Switch/3
